simulink model "Older_model_ contains_ACC"  (R2023b)
settings: Solver=VariableStepAuto  StartTime=0.0  StopTime=30  MaxStep=1e-2  RelTol=1e-3  AbsTol=1e-3
values from neighbouring files (symbols this model uses):
  b = 1.6    [a2024_v2x_matlab_6veh.m]
  m = 2000    [a2024_v2x_matlab_6veh.m]
  mEgo = 1500    [a2024_v2x_matlab_6veh.m]
  sampleTime = 0.1    [a2024_v2x_matlab_6veh.m]    (also in v2x_matlab.m; v2x_matlabV2.m; v2x_matlab_6veh.m; v2x_matlab_R.m)
  t_gap = 1.4    [a2024_v2x_matlab_6veh.m]
  waypoints = [egoWP(:,2) egoWP(:,1), zeroforwp]    [a2024_v2x_matlab_6veh.m]    (also in misc.m = data.data.ActorSpecifications(1,1).Waypoints(:,[1,2]); v2x_matlab.m = data.data.ActorSpecifications(1,1).Waypoints(:,[1,2]); v2x_matlabV2.m = [5 -1.6 0; v2x_matlab_R.m = [5 -1.6 0)
  ZeroActors = struct(     'ActorID',0,     'Position', [1000 1000 1000],      'Velocity', [0 0 0],      'Roll', 0,      'Pitch', 0,      'Yaw', 0,      'AngularVelocity', [0 0 0])    [v2x_matlabV2.m]    (also in v2x_matlab_R.m)
undefined symbols (not defined in the file or in its folder): doppler, driving, n, PredictionHorizon, Ts
libraries: simulink x13, simulink_extras x12, commofdm x10, commdigbbndam3 x10, commchan3 x3, drivingscenarioandsensors x3, mpcadaslib x2, commsink2 x2, vehdynlibdriver x1, dspmathops x1, autolibshared x1
(part 3 of 3)

== matlab function Older_model_ contains_ACC/Vehicle 3/MATLAB Function2 ==
  data: busActors3Test1 input; intVector output int16 size=15; VehicleID input
  events: trigger input RISING_EDGE_EVENT
function intVector = convBus2IntVector(busActors3Test1, VehicleID)

% Data extracted from actorss bus

%ActorId = BusActors1Actors.Actors(ActorID).ActorID(1:1);
numActors = busActors3Test1.NumActors;
time = busActors3Test1.Time;

ActorID = VehicleID;

posX = busActors3Test1.Actors(ActorID).Position(1:1);
posY = busActors3Test1.Actors(ActorID).Position(2:2);
posZ = busActors3Test1.Actors(ActorID).Position(3:3);

vX = busActors3Test1.Actors(ActorID).Velocity(1:1);
vY = busActors3Test1.Actors(ActorID).Velocity(2:2);
vZ = busActors3Test1.Actors(ActorID).Velocity(3:3);

roll = busActors3Test1.Actors(ActorID).Roll(1:1);
pitch = busActors3Test1.Actors(ActorID).Pitch(1:1);
yaw = busActors3Test1.Actors(ActorID).Yaw(1:1);


angularVelocityX = busActors3Test1.Actors(ActorID).AngularVelocity(1:1);
angularVelocityY = busActors3Test1.Actors(ActorID).AngularVelocity(2:2);
angularVelocityZ = busActors3Test1.Actors(ActorID).AngularVelocity(3:3);


% Converting the data

ActorID = int16(ActorID);

posMultip = 10;
posX = int16(round(posMultip*posX));
posY = int16(round(posMultip*posY));
posZ = int16(round(posMultip*posZ));

velMultip = 50;
vX = int16(round(velMultip * vX));
vY = int16(round(velMultip * vY));
vZ = int16(round(velMultip * vZ));

rpyMultip = 50;
roll = int16(round(rpyMultip * roll));
pitch = int16(round(rpyMultip * pitch));
yaw = int16(round(rpyMultip * yaw));

angvelMultip = 50;
angularVelocityX = int16(round(angvelMultip * angularVelocityX));
angularVelocityY = int16(round(angvelMultip * angularVelocityY));
angularVelocityZ = int16(round(angvelMultip * angularVelocityZ));


% Output vector
%zerosVector = zeros(9,1);

intVector = [numActors; time; ActorID; posX; posY; posZ; vX; vY; vZ; roll; pitch; yaw; angularVelocityX; angularVelocityY; angularVelocityZ];
end

== matlab function Older_model_ contains_ACC/Subsystem1/MATLAB Function1 ==
  data: busActors3Test1 input; Actor output int16 size=15; VehicleID input; VehicleData output Bus: Actors; EgoData input Bus: Actors; counter output
  events: trigger input RISING_EDGE_EVENT
function [Actor, VehicleData, counter]  = convBus2IntVector(busActors3Test1, VehicleID, EgoData)

% Data extracted from actorss bus

%ActorId = BusActors1Actors.Actors(ActorID).ActorID(1:1);
numActors = busActors3Test1.NumActors;
%time = busActors3Test1.Time;
time = busActors3Test1.Time;

ActorID = VehicleID;

posX = busActors3Test1.Actors(ActorID).Position(1:1);
posY = busActors3Test1.Actors(ActorID).Position(2:2);
posZ = busActors3Test1.Actors(ActorID).Position(3:3);
vPos = [posX posY posZ];

vX = busActors3Test1.Actors(ActorID).Velocity(1:1);
vY = busActors3Test1.Actors(ActorID).Velocity(2:2);
vZ = busActors3Test1.Actors(ActorID).Velocity(3:3);

roll = busActors3Test1.Actors(ActorID).Roll(1:1);
pitch = busActors3Test1.Actors(ActorID).Pitch(1:1);
yaw = busActors3Test1.Actors(ActorID).Yaw(1:1);


angularVelocityX = busActors3Test1.Actors(ActorID).AngularVelocity(1:1);
angularVelocityY = busActors3Test1.Actors(ActorID).AngularVelocity(2:2);
angularVelocityZ = busActors3Test1.Actors(ActorID).AngularVelocity(3:3);

VehicleData = busActors3Test1.Actors(ActorID);


%% Converting the data

ActorID = int16(ActorID);

posMultip = 10;
posX = int16(round(posMultip*posX));
posY = int16(round(posMultip*posY));
posZ = int16(round(posMultip*posZ));

velMultip = 50;
vX = int16(round(velMultip * vX));
vY = int16(round(velMultip * vY));
vZ = int16(round(velMultip * vZ));

rpyMultip = 50;
roll = int16(round(rpyMultip * roll));
pitch = int16(round(rpyMultip * pitch));
yaw = int16(round(rpyMultip * yaw));

angvelMultip = 50;
angularVelocityX = int16(round(angvelMultip * angularVelocityX));
angularVelocityY = int16(round(angvelMultip * angularVelocityY));
angularVelocityZ = int16(round(angvelMultip * angularVelocityZ));


% Output vector
%zerosVector = zeros(9,1);

intVector = [numActors; time; ActorID; posX; posY; posZ; vX; vY; vZ; roll; pitch; yaw; angularVelocityX; angularVelocityY; angularVelocityZ];



%% Pathloss (freespace)

EgoPos = EgoData.Position;
dist = norm(vPos - EgoPos);

fc = 5.9*10^9;  % Carrier frequency
lambda = physconst('LightSpeed')/fc;

PL = fspl(dist, lambda);

Pt_dBm = 33;    % [dBm] Transmission power; maximum permissible transmit power level
sigma = rand(1) + 3.2;  % [3.7 +- 0.5] Variance of the shadowing effect in the wireless communication channel
                        % shadowing follows a log-normal random distribution
X = randn(1);       % random variable following a normal distribution with mean 0 and standard deviation 1
SH = sigma * X;

Pr = Pt_dBm - PL - SH;

P_SEN = -60;

ZeroActors = int16(zeros(15,1));

persistent prev_value;
if isempty(prev_value)
    prev_value = ZeroActors; % Initialize to a default value
end

if Pr > P_SEN
    Actor = intVector;
    prev_value = intVector;
else
    Actor = prev_value;
end


%% Packet counter
counter = 0;

if (Pr > P_SEN)
    counter = counter + 1;
end


end

== matlab function Older_model_ contains_ACC/Choosing target  ==
  settings: updateMethod=DISCRETE  sampleTime=0.01
  data: ActorsMX input; RelDist output double size=1; RelVel output; EgoData input; EgoVel input
function [RelDist, RelVel] = extractLeadInfo(ActorsMX, EgoData, EgoVel)

ActorID = 1; % Ego vehicle ID
% RelDist = 101;
% RelVel = 101;

%% 1. Actors and Egos positon, yaw, and velocity from the incoming data

threshold_dist = 100; % meter
numColumns = size(ActorsMX, 2);  % = the number of vehicles in the scenario - the ego vehicle

ActorsMXpos = double(ActorsMX(4:6,:));   % extracting only the positions
ActorsMXyaw = double(ActorsMX(12,:));   % extracting only the yaw
%ActorsMxvel = double(ActorsMX(7:9,2:end));

% Extracting the position, velocity and yaw of the ego


EgoPos = (double(EgoData.Position))';
EgoVel = double(EgoData.Velocity)';

EgoPosNorm = norm(double(EgoData.Position));
EgoVelNorm = norm(double(EgoData.Velocity));
 
if EgoVelNorm == 0
    EgoVelNorm = 16;
end
EgoYaw = double(deg2rad(EgoData.Yaw));


%% 2. Create a new matrix to store the filtered columns
filteredActorsMX = NaN(size(ActorsMX));
filteredColumnCount = 0;  % Initialize the count of filtered columns


%% 3. Filter the columns to keep the actor only
egoActoriDist = zeros(1,numColumns); % initialize the distance between ego and lead vehicle
egoActoriYaw = zeros(1,numColumns);  % initialize the yaw differnece between ego and lead vehicle

% disp(EgoPosNorm)
% disp(norm(ActorsMXpos(:, 3)))

for i = 1:numColumns
    egoActoriDist(:,i) = norm(ActorsMXpos(:, i)) - EgoPosNorm;
end
%disp(egoActoriDist)
for i = 1:numColumns
    egoActoriYaw(:,i) = ActorsMXyaw(:,i) - EgoYaw;
end

for i = 1:numColumns
     if ActorsMX(3,i) == 1
        %  (abs(egoActoriDist(:,i)) <= threshold_dist) && ...
        % (abs(egoActoriYaw(:,i)) <= 20)
            
        % If the column meets the criteria, copy it to the new matrix
        filteredColumnCount = filteredColumnCount + 1;
        filteredActorsMX(:, filteredColumnCount) = ActorsMX(:,i);
    end
end

% Remove any columns filled with NaN values in filteredActorsMX
filteredActorsMX = filteredActorsMX(:, ~all(isnan(filteredActorsMX)));
filteredActorsMX(:, ~any(filteredActorsMX)) = [];

persistent prev_vel prev_dist;
if isempty(prev_vel)
    prev_vel = 10; % Initialize to a default value
end
if isempty(prev_dist)
    prev_dist = 10; % Initialize to a default value
end



if ~isempty(filteredActorsMX) 
    LeadPos = filteredActorsMX(4:6,1);
    %LeadPosNorm = norm(LeadPos);
    LeadVel = filteredActorsMX(7:9,1);
    LeadVelNorm = norm(LeadVel);
    %disp(filteredActorsMX(1,:));
    RelDist1 =  norm(LeadPos - EgoPos);
    RelVel1 =  LeadVelNorm - EgoVelNorm;
    if ((-500 <= RelDist1) && (RelDist1 <= 500) && (-200 <= RelVel1) && (RelVel1 <= 200))
        RelDist = RelDist1;
        RelVel = RelVel1;
        prev_vel = RelVel1;
        prev_dist = RelDist1;
    else
        RelDist = prev_dist;
        RelVel = prev_vel;
    end
else
    % Handle the case when filteredActorsMX is empty
    RelDist = prev_dist;
    RelVel = prev_vel;
end



end

== matlab function Older_model_ contains_ACC/channel/MATLAB Function ==
  data: u input; y output
function y = SEN(u)

pow = bandpower(u)
p_sen = -60;

% if pow > p_sen
y = u;
  
end

== matlab function Older_model_ contains_ACC/Subsystem2/MATLAB Function1 ==
  data: busActors3Test1 input; Actor output int16 size=15; VehicleID input; VehicleData output Bus: Actors; EgoData input Bus: Actors; counter output
  events: trigger input RISING_EDGE_EVENT
function [Actor, VehicleData, counter]  = convBus2IntVector(busActors3Test1, VehicleID, EgoData)

% Data extracted from actorss bus

%ActorId = BusActors1Actors.Actors(ActorID).ActorID(1:1);
numActors = busActors3Test1.NumActors;
%time = busActors3Test1.Time;
time = busActors3Test1.Time;

ActorID = VehicleID;

posX = busActors3Test1.Actors(ActorID).Position(1:1);
posY = busActors3Test1.Actors(ActorID).Position(2:2);
posZ = busActors3Test1.Actors(ActorID).Position(3:3);
vPos = [posX posY posZ];

vX = busActors3Test1.Actors(ActorID).Velocity(1:1);
vY = busActors3Test1.Actors(ActorID).Velocity(2:2);
vZ = busActors3Test1.Actors(ActorID).Velocity(3:3);

roll = busActors3Test1.Actors(ActorID).Roll(1:1);
pitch = busActors3Test1.Actors(ActorID).Pitch(1:1);
yaw = busActors3Test1.Actors(ActorID).Yaw(1:1);


angularVelocityX = busActors3Test1.Actors(ActorID).AngularVelocity(1:1);
angularVelocityY = busActors3Test1.Actors(ActorID).AngularVelocity(2:2);
angularVelocityZ = busActors3Test1.Actors(ActorID).AngularVelocity(3:3);

VehicleData = busActors3Test1.Actors(ActorID);


%% Converting the data

ActorID = int16(ActorID);

posMultip = 10;
posX = int16(round(posMultip*posX));
posY = int16(round(posMultip*posY));
posZ = int16(round(posMultip*posZ));

velMultip = 50;
vX = int16(round(velMultip * vX));
vY = int16(round(velMultip * vY));
vZ = int16(round(velMultip * vZ));

rpyMultip = 50;
roll = int16(round(rpyMultip * roll));
pitch = int16(round(rpyMultip * pitch));
yaw = int16(round(rpyMultip * yaw));

angvelMultip = 50;
angularVelocityX = int16(round(angvelMultip * angularVelocityX));
angularVelocityY = int16(round(angvelMultip * angularVelocityY));
angularVelocityZ = int16(round(angvelMultip * angularVelocityZ));


% Output vector
%zerosVector = zeros(9,1);

intVector = [numActors; time; ActorID; posX; posY; posZ; vX; vY; vZ; roll; pitch; yaw; angularVelocityX; angularVelocityY; angularVelocityZ];



%% Pathloss (freespace)

EgoPos = EgoData.Position;
dist = norm(vPos - EgoPos);

fc = 5.9*10^9;  % Carrier frequency
lambda = physconst('LightSpeed')/fc;

PL = fspl(dist, lambda);

Pt_dBm = 33;    % [dBm] Transmission power; maximum permissible transmit power level
sigma = rand(1) + 3.2;  % [3.7 +- 0.5] Variance of the shadowing effect in the wireless communication channel
                        % shadowing follows a log-normal random distribution
X = randn(1);       % random variable following a normal distribution with mean 0 and standard deviation 1
SH = sigma * X;

Pr = Pt_dBm - PL - SH;

P_SEN = -40;

ZeroActors = int16(zeros(15,1));

persistent prev_value;
if isempty(prev_value)
    prev_value = ZeroActors; % Initialize to a default value
end

if Pr > P_SEN
    Actor = intVector;
    prev_value = intVector;
else
    Actor = prev_value;
end


%% Packet counter
counter = 0;

if (Pr > P_SEN)
    counter = counter + 1;
end


end
